simulink model "simulation_vpulse"  (R2022b)
settings: Solver=VariableStepAuto  StartTime=0.0  StopTime=0.35  MaxStep=0.0001  RelTol=1e-3
values from neighbouring files (symbols this model uses):
  C = 40e-3    (= 0.04)    [parameters.m]
  d = 0.302    [parameters.m]
  Lmin = 0.532e-3    (= 0.000532)    [parameters.m]
  m = 8.5e-3    (= 0.0085)    [parameters.m]
  R = 0.7    [parameters.m]
  Rcharge = 20    [parameters.m]
  Tpulse = 18e-3    (= 0.018)    [parameters.m]
  uc0 = 24    [parameters.m]
  uclamp = 67    [parameters.m]
  z0 = -10.5e-3    (= -0.0105)    [parameters.m]
  zs = 7.14e-3    (= 0.00714)    [parameters.m]
settings Model: Creator=Fabian Mink  LastModifiedBy=Fabian Mink

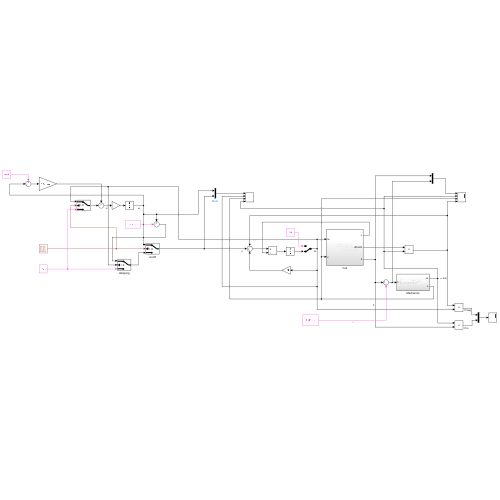
[thumbnail: Simulink's stored preview of the top-level diagram]
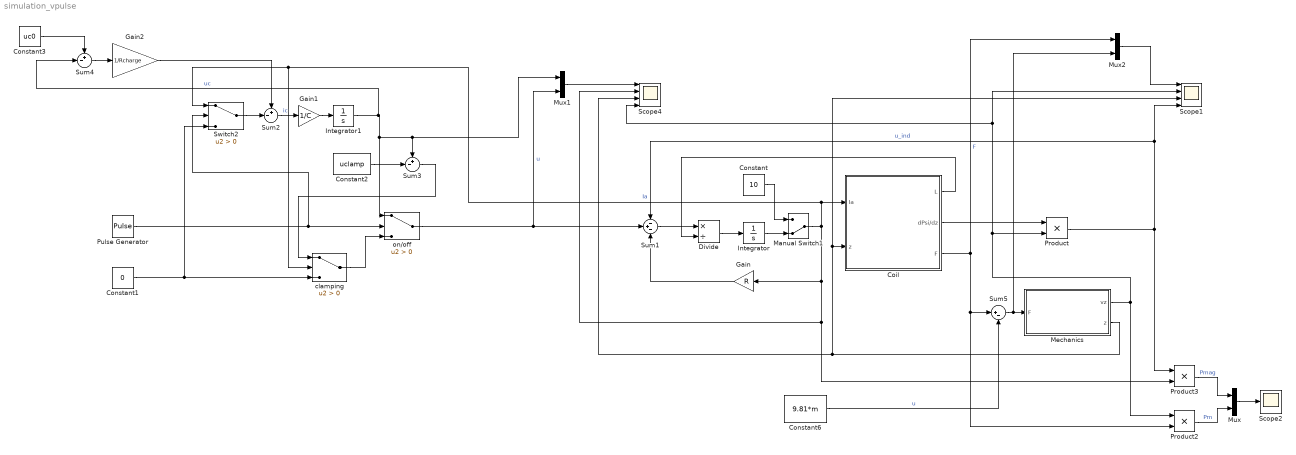
== system simulation_vpulse ==
  Coil : Subsystem
  Constant : Constant  Value=10
  Constant1 : Constant  Value=0
  Constant2 : Constant  Value=uclamp
  Constant3 : Constant  Value=uc0
  Constant6 : Constant  Value=9.81*m
  Divide : Product  Inputs=*/
  Gain : Gain  Gain=R
  Gain1 : Gain  Gain=1/C
  Gain2 : Gain  Gain=1/Rcharge
  Integrator : Integrator
  Integrator1 : Integrator  InitialCondition=uc0
  Manual Switch1 : ManualSwitch  CurrentSetting=0
  Mechanics : Subsystem
  Mux : Mux  Inputs=2
  Mux1 : Mux  Inputs=2
  Mux2 : Mux  Inputs=2
  Product : Product
  Product2 : Product
  Product3 : Product
  Pulse Generator : DiscretePulseGenerator  PulseType=Time based  Period=10  PulseWidth=Tpulse/10*100
  Scope1 : Scope  NumInputPorts=4
  Scope2 : Scope
  Scope4 : Scope  NumInputPorts=4
  Sum1 : Sum  Inputs=-+-
  Sum2 : Sum  Inputs=+-|
  Sum3 : Sum  Inputs=+-|
  Sum4 : Sum  Inputs=+-|
  Sum5 : Sum  Inputs=|+-
  Switch2 : Switch  Criteria=u2 > Threshold  SaturateOnIntegerOverflow=off  InputSameDT=off
  clamping : Switch  Criteria=u2 > Threshold  SaturateOnIntegerOverflow=off  InputSameDT=off
  on/off : Switch  Criteria=u2 > Threshold  SaturateOnIntegerOverflow=off  InputSameDT=off
  wires:
  Manual Switch1/1 -> Scope4/2, Product3/2, Gain/1, clamping/2, Switch2/1, Coil/1(Ia)  "Ia"
  Coil/3(F) -> Sum5/1, Product2/2, Mux2/1  "F"
  Coil/2(dPsi/dz) -> Product/1
  Product/1 -> Product3/1, Scope1/4, Sum1/1  "u_ind"
  Mux/1 -> Scope2/1
  Product3/1 -> Mux/1  "Pmag"
  Product2/1 -> Mux/2  "Pm"
  Constant/1 -> Manual Switch1/1
  Mechanics/1(vz) -> Product2/1, Product/2, Scope1/2, Scope4/4
  Integrator/1 -> Manual Switch1/2
  Divide/1 -> Integrator/1
  Coil/1(L) -> Divide/2
  Sum1/1 -> Divide/1
  Gain/1 -> Sum1/3
  on/off/1 -> Sum1/2, Mux1/2  "u"
  Gain1/1 -> Integrator1/1
  Sum2/1 -> Gain1/1  "ic"
  Pulse Generator/1 -> Switch2/2, on/off/2
  Constant1/1 -> clamping/3, Switch2/3
  Switch2/1 -> Sum2/2
  Integrator1/1 -> Sum4/2, Mux1/1, Sum3/1, on/off/1  "uc"
  clamping/1 -> on/off/3
  Constant2/1 -> Sum3/2
  Sum3/1 -> clamping/1
  Constant3/1 -> Sum4/1
  Sum4/1 -> Gain2/1
  Gain2/1 -> Sum2/1
  Mux1/1 -> Scope4/1
  Sum5/1 -> Mux2/2, Mechanics/1(F)
  Constant6/1 -> Sum5/2  "u"
  Mechanics/2(z) -> Scope4/3, Scope1/3, Coil/2(z)
  Mux2/1 -> Scope1/1

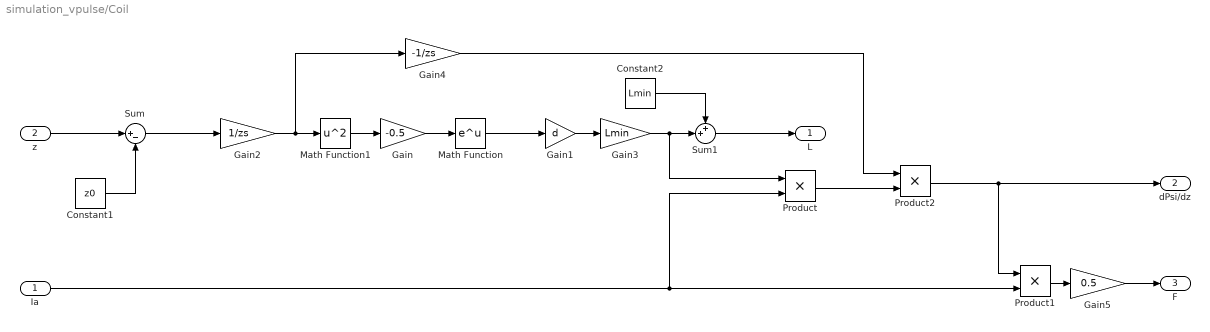
== system simulation_vpulse/Coil ==
  Ia : Inport
  z : Inport  Port=2
  Constant1 : Constant  Value=z0
  Constant2 : Constant  Value=Lmin
  Gain : Gain  Gain=-0.5
  Gain1 : Gain  Gain=d
  Gain2 : Gain  Gain=1/zs
  Gain3 : Gain  Gain=Lmin
  Gain4 : Gain  Gain=-1/zs
  Gain5 : Gain  Gain=0.5
  Math Function : Math
  Math Function1 : Math  Operator=square
  Product : Product
  Product1 : Product
  Product2 : Product
  Sum : Sum  Inputs=|+-
  Sum1 : Sum  Inputs=++|
  L : Outport
  dPsi/dz : Outport  Port=2
  F : Outport  Port=3
  wires:
  Sum/1 -> Gain2/1
  Math Function1/1 -> Gain/1
  Gain2/1 -> Gain4/1, Math Function1/1
  Math Function/1 -> Gain1/1
  Gain/1 -> Math Function/1
  Constant1/1 -> Sum/2
  z/1 -> Sum/1
  Ia/1 -> Product/2, Product1/2
  Product2/1 -> Product1/1, dPsi/dz/1
  Product1/1 -> Gain5/1
  Gain5/1 -> F/1
  Constant2/1 -> Sum1/1
  Gain1/1 -> Gain3/1
  Gain3/1 -> Product/1, Sum1/2
  Sum1/1 -> L/1
  Product/1 -> Product2/2
  Gain4/1 -> Product2/1

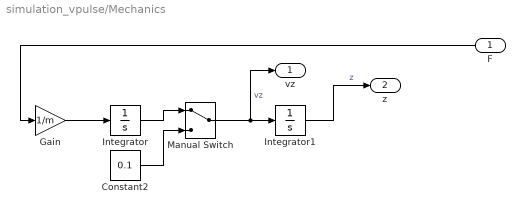
== system simulation_vpulse/Mechanics ==
  F : Inport
  Constant2 : Constant  Value=0.1
  Gain : Gain  Gain=1/m
  Integrator : Integrator
  Integrator1 : Integrator  InitialCondition=-30e-3
  Manual Switch : ManualSwitch
  vz : Outport
  z : Outport  Port=2
  wires:
  Integrator/1 -> Manual Switch/1
  Constant2/1 -> Manual Switch/2
  F/1 -> Gain/1
  Gain/1 -> Integrator/1
  Manual Switch/1 -> vz/1, Integrator1/1  "vz"
  Integrator1/1 -> z/1  "z"
